simulink library "HybridFEMLibrary"  (Simulink 7.0)
undefined symbols (not defined in the file or in its folder): Alpham, DiscIntNeverNeededParam, Elements, gamma1, gamma2, Integrator, Interpolations, sample, SampleRate
(part 1 of 2)
settings Model: Creator=Tommy  LastModifiedBy=Tommy

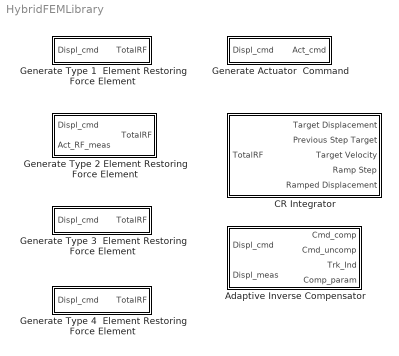
== system HybridFEMLibrary ==
  Adaptive Inverse Compensator : Subsystem
      mask Type: AIC
      mask Description: Adaptive Inverse Compensator produces a compensated command due to actuator delay.  Outputs the compensated and uncompensated response along with a tracking indicator and evolutionary compensation parameter.
  CR Integrator : Subsystem
      mask Type: CR Integrator
      mask Description: CR Integrator for performing the integration of the effective force history to produce the displacement and velocity commands for each time step.  Also combines the restoring force vectors and calculates the next step acceleration.
  Generate Actuator  Command : Subsystem  mask(Generate Actuator Command){id=0}
      mask prompts: id "Element ID"
      mask help:
      | Generates the local actuator command for the element referenced with Element ID
      |
      | Enter the ID for this element corresponding with the input configuration file
  Generate Type 1  Element Restoring Force Element : Subsystem  TreatAsAtomicUnit=on  SystemSampleTime=SampleRate  mask(Generate Type 1 Element Restoring Force){id=32}
      mask prompts: id "Element ID"
      mask help:
      | Generates the Restoring Force vector for a Type 1 Element
      |
      | Enter the ID for this element corresponding with the input configuration file
  Generate Type 2 Element Restoring Force Element : Subsystem  mask(Generate Type 2 Element Restoring Force){id=3, simulation=on}
      mask prompts: id "Element ID"; simulation "Experiment Mode"
      mask help:
      | Generates the Restoring Force vector for a Type 2 Element
      |
      | Enter the ID for this element corresponding with the input configuration file
      |
      | Check the "Experiment Mode" box to activate the Act_RF_meas input.
      | Connect the Actuator Restoring Force feedback to the input.
  Generate Type 3  Element Restoring Force Element : Subsystem  TreatAsAtomicUnit=on  SystemSampleTime=SampleRate  mask(Generate Type 3 Element Restoring Force){id=1}
      mask prompts: id "Element ID"
      mask help:
      | Generates the Restoring Force vector for a Type 3 Element
      |
      | Enter the ID for this element corresponding with the input configuration file
  Generate Type 4  Element Restoring Force Element : Subsystem  TreatAsAtomicUnit=on  SystemSampleTime=SampleRate  mask(Generate Type 4 Element Restoring Force){id=35}
      mask prompts: id "Element ID"
      mask help:
      | Generates the Restoring Force vector for a Type 4 Element
      |
      | Enter the ID for this element corresponding with the input configuration file

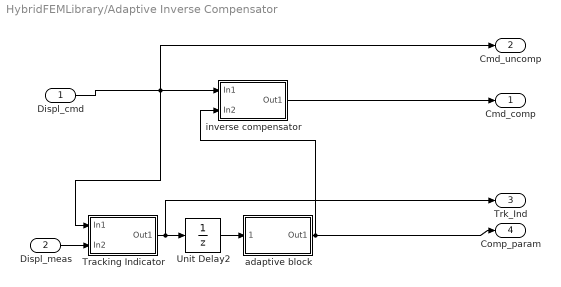
== system HybridFEMLibrary/Adaptive Inverse Compensator ==
  Displ_cmd : Inport  OutDataType=sfix(16)  OutScaling=2^0
  Displ_meas : Inport  Port=2  OutDataType=sfix(16)  OutScaling=2^0
  Tracking Indicator : Subsystem
  Unit Delay2 : UnitDelay  SampleTime=sample
  adaptive block : Subsystem
  inverse compensator : Subsystem
  Cmd_comp : Outport  OutDataType=sfix(16)  OutScaling=2^0
  Cmd_uncomp : Outport  Port=2  OutDataType=sfix(16)  OutScaling=2^0
  Trk_Ind : Outport  Port=3  OutDataType=sfix(16)  OutScaling=2^0
  Comp_param : Outport  Port=4  OutDataType=sfix(16)  OutScaling=2^0
  wires:
  inverse compensator/1(Out1) -> Cmd_comp/1
  adaptive block/1(Out1) -> inverse compensator/2(In2), Comp_param/1
  Tracking Indicator/1(Out1) -> Unit Delay2/1, Trk_Ind/1
  Unit Delay2/1 -> adaptive block/1(indicator)
  Displ_cmd/1 -> Cmd_uncomp/1, inverse compensator/1(In1), Tracking Indicator/1(In1)
  Displ_meas/1 -> Tracking Indicator/2(In2)

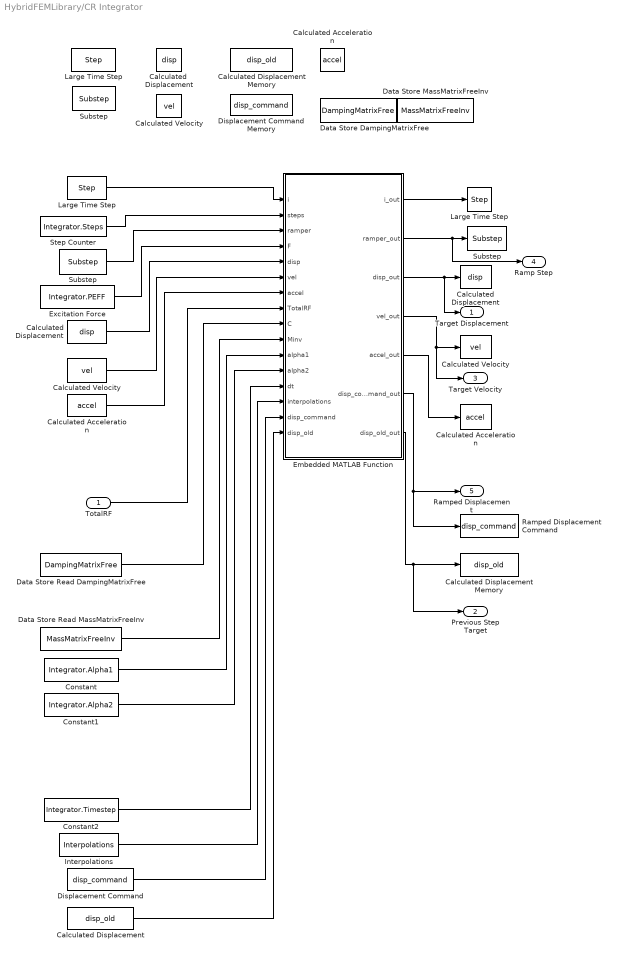
== system HybridFEMLibrary/CR Integrator ==
  TotalRF : Inport  OutDataType=sfix(16)  OutScaling=2^0
  " Calculated Acceleration" : DataStoreWrite  DataStoreName=accel  SampleTime=sample
  " Calculated Displacement" : DataStoreWrite  DataStoreName=disp  SampleTime=sample
  " Calculated Displacement Memory" : DataStoreWrite  DataStoreName=disp_old  SampleTime=sample
  " Calculated Velocity" : DataStoreWrite  DataStoreName=vel  SampleTime=sample
  " Large Time Step" : DataStoreWrite  DataStoreName=Step  SampleTime=sample
  " Substep" : DataStoreWrite  DataStoreName=Substep  SampleTime=sample
  Calculated Acceleration : DataStoreMemory  DataStoreName=accel  InitialValue=Integrator.Acceleration  OutDataType=sfix(16)  OutScaling=2^0
  Calculated Velocity : DataStoreMemory  DataStoreName=vel  InitialValue=Integrator.Velocity  OutDataType=sfix(16)  OutScaling=2^0
  Calculated  Displacement : DataStoreMemory  DataStoreName=disp  InitialValue=Integrator.Displacement  OutDataType=sfix(16)  OutScaling=2^0
  "Calculated Acceleration " : DataStoreRead  DataStoreName=accel  SampleTime=sample
  Calculated Displacement : DataStoreRead  DataStoreName=disp_old  SampleTime=sample
  Calculated Displacement Memory : DataStoreMemory  DataStoreName=disp_old  InitialValue=Integrator.Displacement  OutDataType=sfix(16)  OutScaling=2^0
  "Calculated Displacement " : DataStoreRead  DataStoreName=disp  SampleTime=sample
  "Calculated Velocity " : DataStoreRead  DataStoreName=vel  SampleTime=sample
  Constant : Constant  Value=Integrator.Alpha1  OutDataType=sfix(16)  OutScaling=2^0
  Constant1 : Constant  Value=Integrator.Alpha2  OutDataType=sfix(16)  OutScaling=2^0
  Constant2 : Constant  Value=Integrator.Timestep  OutDataType=sfix(16)  OutScaling=2^0
  Data Store DampingMatrixFree : DataStoreMemory  DataStoreName=DampingMatrixFree  InitialValue=Structure.DampingMatrixFree  OutDataType=sfix(16)  OutScaling=2^0
  Data Store MassMatrixFreeInv : DataStoreMemory  DataStoreName=MassMatrixFreeInv  InitialValue=Structure.MassMatrixFreeInv  OutDataType=sfix(16)  OutScaling=2^0
  Data Store Read DampingMatrixFree : DataStoreRead  DataStoreName=DampingMatrixFree  SampleTime=sample
  Data Store Read MassMatrixFreeInv : DataStoreRead  DataStoreName=MassMatrixFreeInv  SampleTime=sample
  Displacement Command Memory : DataStoreMemory  DataStoreName=disp_command  InitialValue=Integrator.Displacement  OutDataType=sfix(16)  OutScaling=2^0
  "Displacement Command " : DataStoreRead  DataStoreName=disp_command  SampleTime=sample
  Embedded MATLAB Function : Stateflow chart
  Excitation Force : Constant  Value=Integrator.PEFF  OutDataType=sfix(16)  OutScaling=2^0
  Interpolations : Constant  Value=Interpolations  OutDataType=sfix(16)  OutScaling=2^0  SampleTime=sample
  Large Time Step : DataStoreMemory  DataStoreName=Step  OutDataType=sfix(16)  OutScaling=2^0
  "Large Time Step " : DataStoreRead  DataStoreName=Step  SampleTime=sample
  Ramped Displacement Command : DataStoreWrite  DataStoreName=disp_command  SampleTime=sample
  Step Counter : Constant  Value=Integrator.Steps  OutDataType=sfix(16)  OutScaling=2^0  SampleTime=sample
  Substep : DataStoreMemory  DataStoreName=Substep  InitialValue=1  OutDataType=sfix(16)  OutScaling=2^0
  "Substep " : DataStoreRead  DataStoreName=Substep  SampleTime=sample
  Target Displacement : Outport  OutDataType=sfix(16)  OutScaling=2^0
  Previous Step Target : Outport  Port=2  OutDataType=sfix(16)  OutScaling=2^0
  Target Velocity : Outport  Port=3  OutDataType=sfix(16)  OutScaling=2^0
  Ramp Step : Outport  Port=4  OutDataType=sfix(16)  OutScaling=2^0
  Ramped Displacement : Outport  Port=5  OutDataType=sfix(16)  OutScaling=2^0
  wires:
  Excitation Force/1 -> Embedded MATLAB Function/4(F)
  Calculated Displacement/1 -> Embedded MATLAB Function/16(disp_old)
  "Displacement Command "/1 -> Embedded MATLAB Function/15(disp_command)
  "Calculated Acceleration "/1 -> Embedded MATLAB Function/7(accel)
  "Calculated Velocity "/1 -> Embedded MATLAB Function/6(vel)
  "Calculated Displacement "/1 -> Embedded MATLAB Function/5(disp)
  "Substep "/1 -> Embedded MATLAB Function/3(ramper)
  Embedded MATLAB Function/7(disp_old_out) -> Previous Step Target/1, " Calculated Displacement Memory"/1
  Embedded MATLAB Function/5(accel_out) -> " Calculated Acceleration"/1
  Embedded MATLAB Function/3(disp_out) -> " Calculated Displacement"/1, Target Displacement/1
  Embedded MATLAB Function/2(ramper_out) -> Ramp Step/1, " Substep"/1
  Embedded MATLAB Function/1(i_out) -> " Large Time Step"/1
  Constant1/1 -> Embedded MATLAB Function/12(alpha2)
  Constant/1 -> Embedded MATLAB Function/11(alpha1)
  Step Counter/1 -> Embedded MATLAB Function/2(steps)
  Constant2/1 -> Embedded MATLAB Function/13(dt)
  TotalRF/1 -> Embedded MATLAB Function/8(TotalRF)
  Embedded MATLAB Function/6(disp_command_out) -> Ramped Displacement Command/1, Ramped Displacement/1
  Embedded MATLAB Function/4(vel_out) -> " Calculated Velocity"/1, Target Velocity/1
  Interpolations/1 -> Embedded MATLAB Function/14(interpolations)
  Data Store Read MassMatrixFreeInv/1 -> Embedded MATLAB Function/10(Minv)
  Data Store Read DampingMatrixFree/1 -> Embedded MATLAB Function/9(C)
  "Large Time Step "/1 -> Embedded MATLAB Function/1(i)

== system HybridFEMLibrary/Generate Actuator  Command ==
  Displ_cmd : Inport  OutDataType=sfix(16)  OutScaling=2^0
  Generate Actuator Command : Stateflow chart
  Type 2 Element : Subsystem  mask(Element Type 2){id=3}
      mask prompts: id "Element ID:"
      mask help: Enter the ID for this element corresponding with the input configuration file
  Act_cmd : Outport  OutDataType=sfix(16)  OutScaling=2^0
  wires:
  Generate Actuator Command/1(Command) -> Act_cmd/1
  Type 2 Element/1(Element) -> Generate Actuator Command/1(Element)
  Displ_cmd/1 -> Generate Actuator Command/2(Displacement)

== system HybridFEMLibrary/Generate Type 1  Element Restoring Force Element ==
  Displ_cmd : Inport  OutDataType=sfix(16)  OutScaling=2^0
  "Type 1 Element " : Subsystem  mask(Element Type 1){id=id}
      mask prompts: id "Element ID:"
      mask help: Enter the ID for this element corresponding with the input configuration file
  Type 1 Element RF : Stateflow chart  TreatAsAtomicUnit=on  SystemSampleTime=SampleRate
  TotalRF : Outport  OutDataType=sfix(16)  OutScaling=2^0
  wires:
  Type 1 Element RF/1(TotalRF) -> TotalRF/1
  Displ_cmd/1 -> Type 1 Element RF/2(Displacement)
  "Type 1 Element "/1(Element) -> Type 1 Element RF/1(Element)

== system HybridFEMLibrary/Generate Type 2 Element Restoring Force Element ==
  Displ_cmd : Inport  OutDataType=sfix(16)  OutScaling=2^0
  Act_RF_meas : Inport  Port=2  OutDataType=sfix(16)  OutScaling=2^0
  Constant1 : Constant  Value=simulation  OutDataType=sfix(16)  OutScaling=2^0
  Type 2 Element : Subsystem  mask(Element Type 2){id=id}
      mask prompts: id "Element ID:"
      mask help: Enter the ID for this element corresponding with the input configuration file
  Type 2 Element RF : Stateflow chart
  TotalRF : Outport  OutDataType=sfix(16)  OutScaling=2^0
  wires:
  Type 2 Element/1(Element) -> Type 2 Element RF/1(Element)
  Act_RF_meas/1 -> Type 2 Element RF/3(ActuatorRF)
  Type 2 Element RF/1(TotalRF) -> TotalRF/1
  Displ_cmd/1 -> Type 2 Element RF/2(Displacement)
  Constant1/1 -> Type 2 Element RF/4(simulation)

== system HybridFEMLibrary/Generate Type 3  Element Restoring Force Element ==
  Displ_cmd : Inport  OutDataType=sfix(16)  OutScaling=2^0
  "Type 3 Element " : Subsystem  mask(Element Type 3){id=id}
      mask prompts: id "Element ID:"
      mask help: Enter the ID for this element corresponding with the input configuration file
  Type 3 Element RF : Stateflow chart  TreatAsAtomicUnit=on  SystemSampleTime=SampleRate
  TotalRF : Outport  OutDataType=sfix(16)  OutScaling=2^0
  wires:
  Displ_cmd/1 -> Type 3 Element RF/6(Displacement)
  "Type 3 Element "/1(Element) -> Type 3 Element RF/1(Element)
  Type 3 Element RF/1(TotalRF) -> TotalRF/1
  "Type 3 Element "/2(a1) -> Type 3 Element RF/2(a1)
  "Type 3 Element "/3(a2) -> Type 3 Element RF/3(a2)
  "Type 3 Element "/4(pmx) -> Type 3 Element RF/4(pmx)
  "Type 3 Element "/5(bmy) -> Type 3 Element RF/5(bmy_init)

== system HybridFEMLibrary/Generate Type 4  Element Restoring Force Element ==
  Displ_cmd : Inport  OutDataType=sfix(16)  OutScaling=2^0
  "Type 4 Element " : Subsystem  mask(Element Type 4){id=id}
      mask prompts: id "Element ID:"
      mask help: Enter the ID for this element corresponding with the input configuration file
  Type 4 Element RF : Stateflow chart  TreatAsAtomicUnit=on  SystemSampleTime=SampleRate
  TotalRF : Outport  OutDataType=sfix(16)  OutScaling=2^0
  wires:
  "Type 4 Element "/1(Element) -> Type 4 Element RF/1(Element)
  Type 4 Element RF/1(TotalRF) -> TotalRF/1
  Displ_cmd/1 -> Type 4 Element RF/2(Displacement)

== system HybridFEMLibrary/Adaptive Inverse Compensator/Tracking Indicator ==
  note: dc
  note: dm
  note: A
  note: TA
  note: TI
  In1 : Inport  OutDataType=sfix(16)  OutScaling=2^0
  In2 : Inport  Port=2  OutDataType=sfix(16)  OutScaling=2^0
  A : Subsystem
  Gain : Gain  Gain=0.5  ParameterDataType=sfix(16)  ParameterScaling=2^0  OutDataType=sfix(16)  OutScaling=2^0
  Scope : Scope
      settings: SaveName=ScopeData4
  Sum : Sum  Inputs=|+-  OutDataType=sfix(16)  OutScaling=2^0
  TA : Subsystem
  Out1 : Outport  OutDataType=sfix(16)  OutScaling=2^0
  wires:
  In2/1 -> A/2(In2), TA/2(In2)
  In1/1 -> A/1(In1), TA/1(In1)
  TA/1(Out1) -> Sum/2
  A/1(Out1) -> Sum/1
  Sum/1 -> Gain/1
  Gain/1 -> Out1/1, Scope/1

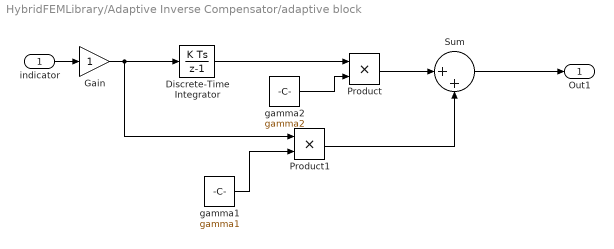
== system HybridFEMLibrary/Adaptive Inverse Compensator/adaptive block ==
  indicator : Inport  OutDataType=sfix(16)  OutScaling=2^0
  Discrete-Time Integrator : DiscreteIntegrator  SampleTime=sample  OutDataType=sfix(16)  OutScaling=2^0  ICPrevOutput=DiscIntNeverNeededParam  ICPrevScaledInput=DiscIntNeverNeededParam
  Gain : Gain  ParameterDataType=sfix(16)  ParameterScaling=2^0  OutDataType=sfix(16)  OutScaling=2^0
  Product : Product  OutDataType=sfix(16)  OutScaling=2^0  RndMeth=Zero
  Product1 : Product  OutDataType=sfix(16)  OutScaling=2^0  RndMeth=Zero
  Sum : Sum  Inputs=|++  OutDataType=sfix(16)  OutScaling=2^0
  gamma1 : Constant  Value=gamma1  OutDataType=sfix(16)  OutScaling=2^0
  gamma2 : Constant  Value=gamma2  OutDataType=sfix(16)  OutScaling=2^0
  Out1 : Outport  OutDataType=sfix(16)  OutScaling=2^0
  wires:
  Discrete-Time Integrator/1 -> Product/1
  gamma2/1 -> Product/2
  gamma1/1 -> Product1/2
  Product/1 -> Sum/1
  Sum/1 -> Out1/1
  indicator/1 -> Gain/1
  Product1/1 -> Sum/2
  Gain/1 -> Discrete-Time Integrator/1, Product1/1

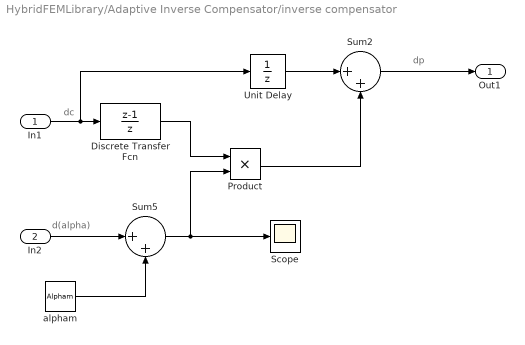
== system HybridFEMLibrary/Adaptive Inverse Compensator/inverse compensator ==
  note: dp
  note: d(alpha)
  note: dc
  In1 : Inport  OutDataType=sfix(16)  OutScaling=2^0
  In2 : Inport  Port=2  OutDataType=sfix(16)  OutScaling=2^0
  Discrete Transfer Fcn : DiscreteTransferFcn  Numerator=[1 -1]  Denominator=[1 0]  SampleTime=sample
  Product : Product  OutDataType=sfix(16)  OutScaling=2^0  RndMeth=Zero
  Scope : Scope
  Sum2 : Sum  Inputs=|++  OutDataType=sfix(16)  OutScaling=2^0
  Sum5 : Sum  Inputs=|++  OutDataType=sfix(16)  OutScaling=2^0
  Unit Delay : UnitDelay  SampleTime=sample
  alpham : Constant  Value=Alpham  OutDataType=sfix(16)  OutScaling=2^0
  Out1 : Outport  OutDataType=sfix(16)  OutScaling=2^0
  wires:
  Sum2/1 -> Out1/1
  Product/1 -> Sum2/2
  Unit Delay/1 -> Sum2/1
  Sum5/1 -> Scope/1, Product/2
  Discrete Transfer Fcn/1 -> Product/1
  alpham/1 -> Sum5/2
  In2/1 -> Sum5/1
  In1/1 -> Unit Delay/1, Discrete Transfer Fcn/1

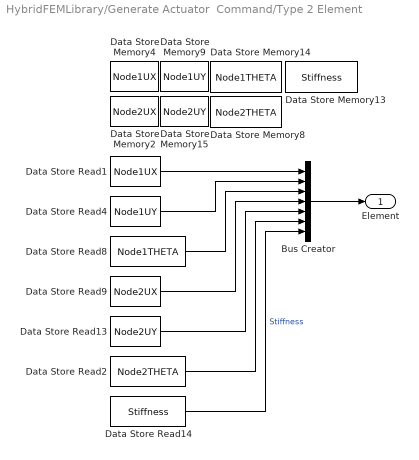
== system HybridFEMLibrary/Generate Actuator  Command/Type 2 Element ==
  Bus Creator : BusCreator  Inputs=7
  Data Store Memory13 : DataStoreMemory  DataStoreName=Stiffness  InitialValue=Elements{id}.Stiffness  OutDataType=sfix(16)  OutScaling=2^0
  Data Store Memory14 : DataStoreMemory  DataStoreName=Node1THETA  InitialValue=Elements{id}.Nodes(1).THETA  OutDataType=sfix(16)  OutScaling=2^0
  Data Store Memory15 : DataStoreMemory  DataStoreName=Node2UY  InitialValue=Elements{id}.Nodes(2).UY  OutDataType=sfix(16)  OutScaling=2^0
  Data Store Memory2 : DataStoreMemory  DataStoreName=Node2UX  InitialValue=Elements{id}.Nodes(2).UX  OutDataType=sfix(16)  OutScaling=2^0
  Data Store Memory4 : DataStoreMemory  DataStoreName=Node1UX  InitialValue=Elements{id}.Nodes(1).UX  OutDataType=sfix(16)  OutScaling=2^0
  Data Store Memory8 : DataStoreMemory  DataStoreName=Node2THETA  InitialValue=Elements{id}.Nodes(2).THETA  OutDataType=sfix(16)  OutScaling=2^0
  Data Store Memory9 : DataStoreMemory  DataStoreName=Node1UY  InitialValue=Elements{id}.Nodes(1).UY  OutDataType=sfix(16)  OutScaling=2^0
  Data Store Read1 : DataStoreRead  DataStoreName=Node1UX  SampleTime=-1
  Data Store Read13 : DataStoreRead  DataStoreName=Node2UY  SampleTime=-1
  Data Store Read14 : DataStoreRead  DataStoreName=Stiffness  SampleTime=-1
  Data Store Read2 : DataStoreRead  DataStoreName=Node2THETA  SampleTime=-1
  Data Store Read4 : DataStoreRead  DataStoreName=Node1UY  SampleTime=-1
  Data Store Read8 : DataStoreRead  DataStoreName=Node1THETA  SampleTime=-1
  Data Store Read9 : DataStoreRead  DataStoreName=Node2UX  SampleTime=-1
  Element : Outport  OutDataType=sfix(16)  OutScaling=2^0
  wires:
  Bus Creator/1 -> Element/1
  Data Store Read14/1 -> Bus Creator/7  "Stiffness"
  Data Store Read2/1 -> Bus Creator/6
  Data Store Read13/1 -> Bus Creator/5
  Data Store Read9/1 -> Bus Creator/4
  Data Store Read8/1 -> Bus Creator/3
  Data Store Read4/1 -> Bus Creator/2
  Data Store Read1/1 -> Bus Creator/1

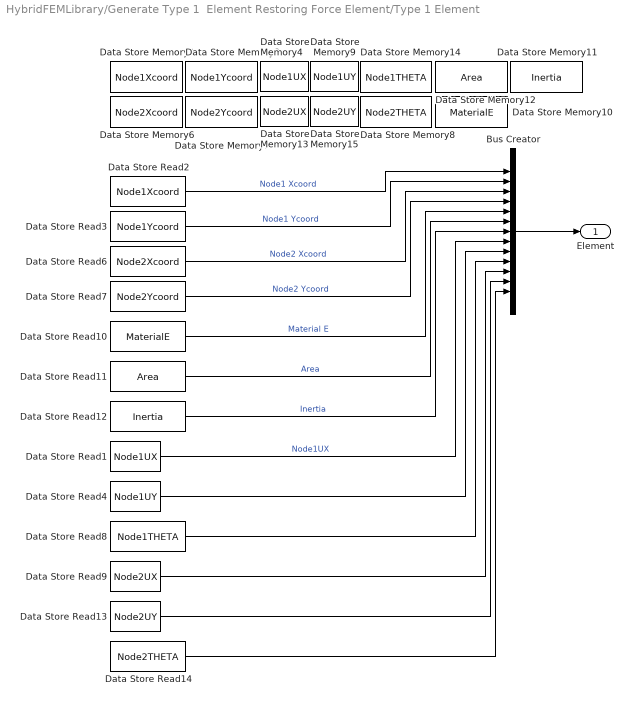
== system HybridFEMLibrary/Generate Type 1  Element Restoring Force Element/Type 1 Element  ==
  Bus Creator : BusCreator  Inputs=13
  Data Store Memory10 : DataStoreMemory  DataStoreName=MaterialE  InitialValue=Elements{id}.Material(1).E  OutDataType=sfix(16)  OutScaling=2^0
  Data Store Memory11 : DataStoreMemory  DataStoreName=Inertia  InitialValue=Elements{id}.Inertia  OutDataType=sfix(16)  OutScaling=2^0
  Data Store Memory12 : DataStoreMemory  DataStoreName=Area  InitialValue=Elements{id}.Area  OutDataType=sfix(16)  OutScaling=2^0
  Data Store Memory13 : DataStoreMemory  DataStoreName=Node2UX  InitialValue=Elements{id}.Nodes(2).UX  OutDataType=sfix(16)  OutScaling=2^0
  Data Store Memory14 : DataStoreMemory  DataStoreName=Node1THETA  InitialValue=Elements{id}.Nodes(1).THETA  OutDataType=sfix(16)  OutScaling=2^0
  Data Store Memory15 : DataStoreMemory  DataStoreName=Node2UY  InitialValue=Elements{id}.Nodes(2).UY  OutDataType=sfix(16)  OutScaling=2^0
  Data Store Memory2 : DataStoreMemory  DataStoreName=Node1Xcoord  InitialValue=Elements{id}.Nodes(1).Xcoord  OutDataType=sfix(16)  OutScaling=2^0
  Data Store Memory3 : DataStoreMemory  DataStoreName=Node1Ycoord  InitialValue=Elements{id}.Nodes(1).Ycoord  OutDataType=sfix(16)  OutScaling=2^0
  Data Store Memory4 : DataStoreMemory  DataStoreName=Node1UX  InitialValue=Elements{id}.Nodes(1).UX  OutDataType=sfix(16)  OutScaling=2^0
  Data Store Memory6 : DataStoreMemory  DataStoreName=Node2Xcoord  InitialValue=Elements{id}.Nodes(2).Xcoord  OutDataType=sfix(16)  OutScaling=2^0
  Data Store Memory7 : DataStoreMemory  DataStoreName=Node2Ycoord  InitialValue=Elements{id}.Nodes(2).Ycoord  OutDataType=sfix(16)  OutScaling=2^0
  Data Store Memory8 : DataStoreMemory  DataStoreName=Node2THETA  InitialValue=Elements{id}.Nodes(2).THETA  OutDataType=sfix(16)  OutScaling=2^0
  Data Store Memory9 : DataStoreMemory  DataStoreName=Node1UY  InitialValue=Elements{id}.Nodes(1).UY  OutDataType=sfix(16)  OutScaling=2^0
  Data Store Read1 : DataStoreRead  DataStoreName=Node1UX  SampleTime=-1
  Data Store Read10 : DataStoreRead  DataStoreName=MaterialE  SampleTime=-1
  Data Store Read11 : DataStoreRead  DataStoreName=Area  SampleTime=-1
  Data Store Read12 : DataStoreRead  DataStoreName=Inertia  SampleTime=-1
  Data Store Read13 : DataStoreRead  DataStoreName=Node2UY  SampleTime=-1
  Data Store Read14 : DataStoreRead  DataStoreName=Node2THETA  SampleTime=-1
  Data Store Read2 : DataStoreRead  DataStoreName=Node1Xcoord  SampleTime=-1
  Data Store Read3 : DataStoreRead  DataStoreName=Node1Ycoord  SampleTime=-1
  Data Store Read4 : DataStoreRead  DataStoreName=Node1UY  SampleTime=-1
  Data Store Read6 : DataStoreRead  DataStoreName=Node2Xcoord  SampleTime=-1
  Data Store Read7 : DataStoreRead  DataStoreName=Node2Ycoord  SampleTime=-1
  Data Store Read8 : DataStoreRead  DataStoreName=Node1THETA  SampleTime=-1
  Data Store Read9 : DataStoreRead  DataStoreName=Node2UX  SampleTime=-1
  Element : Outport  OutDataType=sfix(16)  OutScaling=2^0
  wires:
  Bus Creator/1 -> Element/1
  Data Store Read12/1 -> Bus Creator/7  "Inertia"
  Data Store Read11/1 -> Bus Creator/6  "Area"
  Data Store Read10/1 -> Bus Creator/5  "Material E"
  Data Store Read7/1 -> Bus Creator/4  "Node2 Ycoord"
  Data Store Read6/1 -> Bus Creator/3  "Node2 Xcoord"
  Data Store Read3/1 -> Bus Creator/2  "Node1 Ycoord"
  Data Store Read2/1 -> Bus Creator/1  "Node1 Xcoord"
  Data Store Read1/1 -> Bus Creator/8  "Node1UX"
  Data Store Read4/1 -> Bus Creator/9
  Data Store Read8/1 -> Bus Creator/10
  Data Store Read9/1 -> Bus Creator/11
  Data Store Read13/1 -> Bus Creator/12
  Data Store Read14/1 -> Bus Creator/13

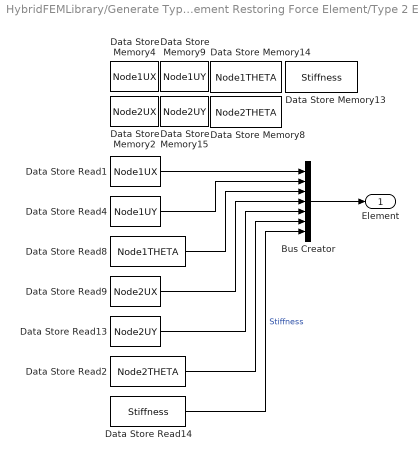
== system HybridFEMLibrary/Generate Type 2 Element Restoring Force Element/Type 2 Element ==
  Bus Creator : BusCreator  Inputs=7
  Data Store Memory13 : DataStoreMemory  DataStoreName=Stiffness  InitialValue=Elements{id}.Stiffness  OutDataType=sfix(16)  OutScaling=2^0
  Data Store Memory14 : DataStoreMemory  DataStoreName=Node1THETA  InitialValue=Elements{id}.Nodes(1).THETA  OutDataType=sfix(16)  OutScaling=2^0
  Data Store Memory15 : DataStoreMemory  DataStoreName=Node2UY  InitialValue=Elements{id}.Nodes(2).UY  OutDataType=sfix(16)  OutScaling=2^0
  Data Store Memory2 : DataStoreMemory  DataStoreName=Node2UX  InitialValue=Elements{id}.Nodes(2).UX  OutDataType=sfix(16)  OutScaling=2^0
  Data Store Memory4 : DataStoreMemory  DataStoreName=Node1UX  InitialValue=Elements{id}.Nodes(1).UX  OutDataType=sfix(16)  OutScaling=2^0
  Data Store Memory8 : DataStoreMemory  DataStoreName=Node2THETA  InitialValue=Elements{id}.Nodes(2).THETA  OutDataType=sfix(16)  OutScaling=2^0
  Data Store Memory9 : DataStoreMemory  DataStoreName=Node1UY  InitialValue=Elements{id}.Nodes(1).UY  OutDataType=sfix(16)  OutScaling=2^0
  Data Store Read1 : DataStoreRead  DataStoreName=Node1UX  SampleTime=-1
  Data Store Read13 : DataStoreRead  DataStoreName=Node2UY  SampleTime=-1
  Data Store Read14 : DataStoreRead  DataStoreName=Stiffness  SampleTime=-1
  Data Store Read2 : DataStoreRead  DataStoreName=Node2THETA  SampleTime=-1
  Data Store Read4 : DataStoreRead  DataStoreName=Node1UY  SampleTime=-1
  Data Store Read8 : DataStoreRead  DataStoreName=Node1THETA  SampleTime=-1
  Data Store Read9 : DataStoreRead  DataStoreName=Node2UX  SampleTime=-1
  Element : Outport  OutDataType=sfix(16)  OutScaling=2^0
  wires:
  Data Store Read1/1 -> Bus Creator/1
  Data Store Read4/1 -> Bus Creator/2
  Data Store Read8/1 -> Bus Creator/3
  Data Store Read9/1 -> Bus Creator/4
  Data Store Read13/1 -> Bus Creator/5
  Data Store Read2/1 -> Bus Creator/6
  Data Store Read14/1 -> Bus Creator/7  "Stiffness"
  Bus Creator/1 -> Element/1

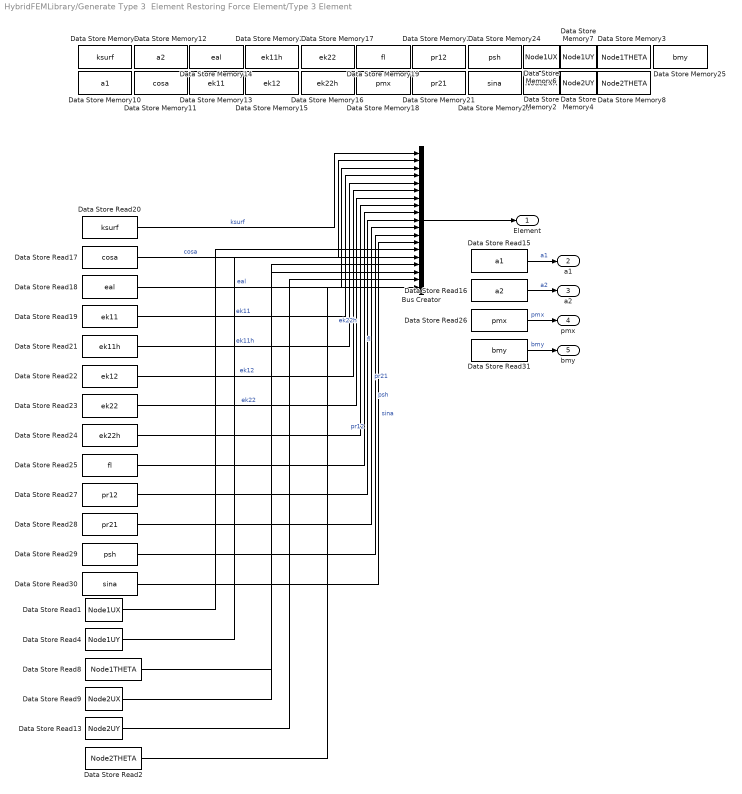
== system HybridFEMLibrary/Generate Type 3  Element Restoring Force Element/Type 3 Element  ==
  Bus Creator : BusCreator  Inputs=19
  Data Store Memory10 : DataStoreMemory  DataStoreName=a1  InitialValue=Elements{id}.a1  OutDataType=sfix(16)  OutScaling=2^0
  Data Store Memory11 : DataStoreMemory  DataStoreName=cosa  InitialValue=Elements{id}.cosa  OutDataType=sfix(16)  OutScaling=2^0
  Data Store Memory12 : DataStoreMemory  DataStoreName=a2  InitialValue=Elements{id}.a2  OutDataType=sfix(16)  OutScaling=2^0
  Data Store Memory13 : DataStoreMemory  DataStoreName=ek11  InitialValue=Elements{id}.ek11  OutDataType=sfix(16)  OutScaling=2^0
  Data Store Memory14 : DataStoreMemory  DataStoreName=eal  InitialValue=Elements{id}.eal  OutDataType=sfix(16)  OutScaling=2^0
  Data Store Memory15 : DataStoreMemory  DataStoreName=ek12  InitialValue=Elements{id}.ek12  OutDataType=sfix(16)  OutScaling=2^0
  Data Store Memory16 : DataStoreMemory  DataStoreName=ek22h  InitialValue=Elements{id}.ek22h  OutDataType=sfix(16)  OutScaling=2^0
  Data Store Memory17 : DataStoreMemory  DataStoreName=ek22  InitialValue=Elements{id}.ek22  OutDataType=sfix(16)  OutScaling=2^0
  Data Store Memory18 : DataStoreMemory  DataStoreName=pmx  InitialValue=Elements{id}.pmx  OutDataType=sfix(16)  OutScaling=2^0
  Data Store Memory19 : DataStoreMemory  DataStoreName=fl  InitialValue=Elements{id}.fl  OutDataType=sfix(16)  OutScaling=2^0
  Data Store Memory2 : DataStoreMemory  DataStoreName=Node2UX  InitialValue=Elements{id}.Nodes(2).UX  OutDataType=sfix(16)  OutScaling=2^0
  Data Store Memory20 : DataStoreMemory  DataStoreName=ek11h  InitialValue=Elements{id}.ek11h  OutDataType=sfix(16)  OutScaling=2^0
  Data Store Memory21 : DataStoreMemory  DataStoreName=pr21  InitialValue=Elements{id}.pr21  OutDataType=sfix(16)  OutScaling=2^0
  Data Store Memory22 : DataStoreMemory  DataStoreName=pr12  InitialValue=Elements{id}.pr12  OutDataType=sfix(16)  OutScaling=2^0
  Data Store Memory23 : DataStoreMemory  DataStoreName=sina  InitialValue=Elements{id}.sina  OutDataType=sfix(16)  OutScaling=2^0
  Data Store Memory24 : DataStoreMemory  DataStoreName=psh  InitialValue=Elements{id}.psh  OutDataType=sfix(16)  OutScaling=2^0
  Data Store Memory25 : DataStoreMemory  DataStoreName=bmy  InitialValue=Elements{id}.bmy  OutDataType=sfix(16)  OutScaling=2^0
  Data Store Memory3 : DataStoreMemory  DataStoreName=Node1THETA  InitialValue=Elements{id}.Nodes(1).THETA  OutDataType=sfix(16)  OutScaling=2^0
  Data Store Memory4 : DataStoreMemory  DataStoreName=Node2UY  InitialValue=Elements{id}.Nodes(2).UY  OutDataType=sfix(16)  OutScaling=2^0
  Data Store Memory6 : DataStoreMemory  DataStoreName=Node1UX  InitialValue=Elements{id}.Nodes(1).UX  OutDataType=sfix(16)  OutScaling=2^0
  Data Store Memory7 : DataStoreMemory  DataStoreName=Node1UY  InitialValue=Elements{id}.Nodes(1).UY  OutDataType=sfix(16)  OutScaling=2^0
  Data Store Memory8 : DataStoreMemory  DataStoreName=Node2THETA  InitialValue=Elements{id}.Nodes(2).THETA  OutDataType=sfix(16)  OutScaling=2^0
  Data Store Memory9 : DataStoreMemory  DataStoreName=ksurf  InitialValue=Elements{id}.ksurf  OutDataType=sfix(16)  OutScaling=2^0
  Data Store Read1 : DataStoreRead  DataStoreName=Node1UX  SampleTime=-1
  Data Store Read13 : DataStoreRead  DataStoreName=Node2UY  SampleTime=-1
  Data Store Read15 : DataStoreRead  DataStoreName=a1  SampleTime=-1
  Data Store Read16 : DataStoreRead  DataStoreName=a2  SampleTime=-1
  Data Store Read17 : DataStoreRead  DataStoreName=cosa  SampleTime=-1
  Data Store Read18 : DataStoreRead  DataStoreName=eal  SampleTime=-1
  Data Store Read19 : DataStoreRead  DataStoreName=ek11  SampleTime=-1
  Data Store Read2 : DataStoreRead  DataStoreName=Node2THETA  SampleTime=-1
  Data Store Read20 : DataStoreRead  DataStoreName=ksurf  SampleTime=-1
  Data Store Read21 : DataStoreRead  DataStoreName=ek11h  SampleTime=-1
  Data Store Read22 : DataStoreRead  DataStoreName=ek12  SampleTime=-1
  Data Store Read23 : DataStoreRead  DataStoreName=ek22  SampleTime=-1
  Data Store Read24 : DataStoreRead  DataStoreName=ek22h  SampleTime=-1
  Data Store Read25 : DataStoreRead  DataStoreName=fl  SampleTime=-1
  Data Store Read26 : DataStoreRead  DataStoreName=pmx  SampleTime=-1
  Data Store Read27 : DataStoreRead  DataStoreName=pr12  SampleTime=-1
  Data Store Read28 : DataStoreRead  DataStoreName=pr21  SampleTime=-1
  Data Store Read29 : DataStoreRead  DataStoreName=psh  SampleTime=-1
  Data Store Read30 : DataStoreRead  DataStoreName=sina  SampleTime=-1
  Data Store Read31 : DataStoreRead  DataStoreName=bmy  SampleTime=-1
  Data Store Read4 : DataStoreRead  DataStoreName=Node1UY  SampleTime=-1
  Data Store Read8 : DataStoreRead  DataStoreName=Node1THETA  SampleTime=-1
  Data Store Read9 : DataStoreRead  DataStoreName=Node2UX  SampleTime=-1
  Element : Outport  OutDataType=sfix(16)  OutScaling=2^0
  a1 : Outport  Port=2  OutDataType=sfix(16)  OutScaling=2^0
  a2 : Outport  Port=3  OutDataType=sfix(16)  OutScaling=2^0
  pmx : Outport  Port=4  OutDataType=sfix(16)  OutScaling=2^0
  bmy : Outport  Port=5  OutDataType=sfix(16)  OutScaling=2^0
  wires:
  Data Store Read31/1 -> bmy/1  "bmy"
  Data Store Read26/1 -> pmx/1  "pmx"
  Data Store Read16/1 -> a2/1  "a2"
  Data Store Read15/1 -> a1/1  "a1"
  Data Store Read30/1 -> Bus Creator/13  "sina"
  Data Store Read29/1 -> Bus Creator/12  "psh"
  Data Store Read28/1 -> Bus Creator/11  "pr21"
  Data Store Read27/1 -> Bus Creator/10  "pr12"
  Data Store Read25/1 -> Bus Creator/9  "fl"
  Data Store Read24/1 -> Bus Creator/8  "ek22h"
  Data Store Read23/1 -> Bus Creator/7  "ek22"
  Data Store Read22/1 -> Bus Creator/6  "ek12"
  Data Store Read21/1 -> Bus Creator/5  "ek11h"
  Data Store Read19/1 -> Bus Creator/4  "ek11"
  Data Store Read18/1 -> Bus Creator/3  "eal"
  Data Store Read17/1 -> Bus Creator/2  "cosa"
  Data Store Read20/1 -> Bus Creator/1  "ksurf"
  Bus Creator/1 -> Element/1
  Data Store Read1/1 -> Bus Creator/14
  Data Store Read4/1 -> Bus Creator/15
  Data Store Read8/1 -> Bus Creator/16
  Data Store Read9/1 -> Bus Creator/17
  Data Store Read13/1 -> Bus Creator/18
  Data Store Read2/1 -> Bus Creator/19

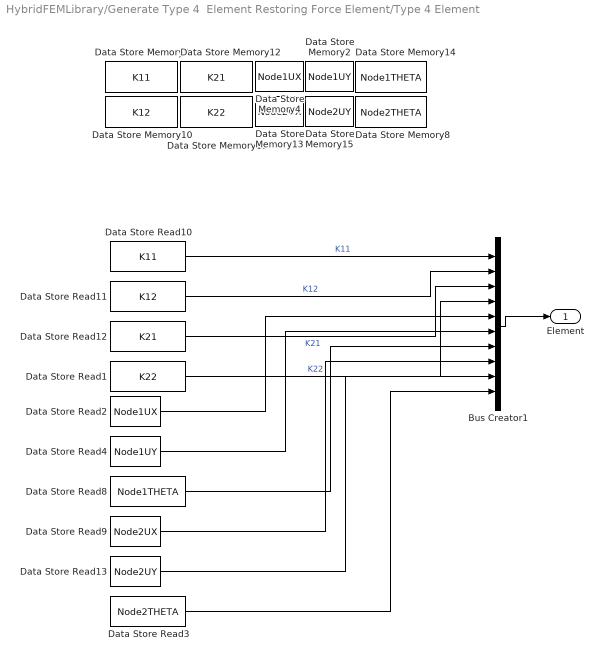
== system HybridFEMLibrary/Generate Type 4  Element Restoring Force Element/Type 4 Element  ==
  Bus Creator1 : BusCreator  Inputs=10
  Data Store Memory10 : DataStoreMemory  DataStoreName=K12  InitialValue=Elements{id}.K12  OutDataType=sfix(16)  OutScaling=2^0
  Data Store Memory11 : DataStoreMemory  DataStoreName=K22  InitialValue=Elements{id}.K22  OutDataType=sfix(16)  OutScaling=2^0
  Data Store Memory12 : DataStoreMemory  DataStoreName=K21  InitialValue=Elements{id}.K21  OutDataType=sfix(16)  OutScaling=2^0
  Data Store Memory13 : DataStoreMemory  DataStoreName=Node2UX  InitialValue=Elements{id}.Nodes(2).UX  OutDataType=sfix(16)  OutScaling=2^0
  Data Store Memory14 : DataStoreMemory  DataStoreName=Node1THETA  InitialValue=Elements{id}.Nodes(1).THETA  OutDataType=sfix(16)  OutScaling=2^0
  Data Store Memory15 : DataStoreMemory  DataStoreName=Node2UY  InitialValue=Elements{id}.Nodes(2).UY  OutDataType=sfix(16)  OutScaling=2^0
  Data Store Memory2 : DataStoreMemory  DataStoreName=Node1UY  InitialValue=Elements{id}.Nodes(1).UY  OutDataType=sfix(16)  OutScaling=2^0
  Data Store Memory4 : DataStoreMemory  DataStoreName=Node1UX  InitialValue=Elements{id}.Nodes(1).UX  OutDataType=sfix(16)  OutScaling=2^0
  Data Store Memory8 : DataStoreMemory  DataStoreName=Node2THETA  InitialValue=Elements{id}.Nodes(2).THETA  OutDataType=sfix(16)  OutScaling=2^0
  Data Store Memory9 : DataStoreMemory  DataStoreName=K11  InitialValue=Elements{id}.K11  OutDataType=sfix(16)  OutScaling=2^0
  Data Store Read1 : DataStoreRead  DataStoreName=K22  SampleTime=-1
  Data Store Read10 : DataStoreRead  DataStoreName=K11  SampleTime=-1
  Data Store Read11 : DataStoreRead  DataStoreName=K12  SampleTime=-1
  Data Store Read12 : DataStoreRead  DataStoreName=K21  SampleTime=-1
  Data Store Read13 : DataStoreRead  DataStoreName=Node2UY  SampleTime=-1
  Data Store Read2 : DataStoreRead  DataStoreName=Node1UX  SampleTime=-1
  Data Store Read3 : DataStoreRead  DataStoreName=Node2THETA  SampleTime=-1
  Data Store Read4 : DataStoreRead  DataStoreName=Node1UY  SampleTime=-1
  Data Store Read8 : DataStoreRead  DataStoreName=Node1THETA  SampleTime=-1
  Data Store Read9 : DataStoreRead  DataStoreName=Node2UX  SampleTime=-1
  Element : Outport  OutDataType=sfix(16)  OutScaling=2^0
  wires:
  Data Store Read3/1 -> Bus Creator1/10
  Data Store Read13/1 -> Bus Creator1/9
  Data Store Read9/1 -> Bus Creator1/8
  Data Store Read8/1 -> Bus Creator1/7
  Data Store Read4/1 -> Bus Creator1/6
  Data Store Read2/1 -> Bus Creator1/5
  Bus Creator1/1 -> Element/1
  Data Store Read10/1 -> Bus Creator1/1  "K11"
  Data Store Read11/1 -> Bus Creator1/2  "K12"
  Data Store Read12/1 -> Bus Creator1/3  "K21"
  Data Store Read1/1 -> Bus Creator1/4  "K22"

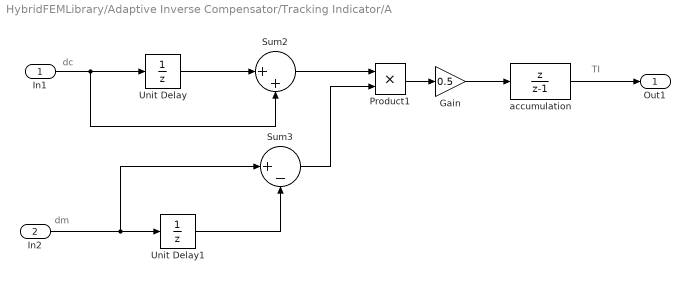
== system HybridFEMLibrary/Adaptive Inverse Compensator/Tracking Indicator/A ==
  note: dc
  note: dm
  note: TI
  In1 : Inport  OutDataType=sfix(16)  OutScaling=2^0
  In2 : Inport  Port=2  OutDataType=sfix(16)  OutScaling=2^0
  Gain : Gain  Gain=0.5  ParameterDataType=sfix(16)  ParameterScaling=2^0  OutDataType=sfix(16)  OutScaling=2^0
  Product1 : Product  OutDataType=sfix(16)  OutScaling=2^0  RndMeth=Zero
  Sum2 : Sum  Inputs=|++  OutDataType=sfix(16)  OutScaling=2^0
  Sum3 : Sum  Inputs=|+-  OutDataType=sfix(16)  OutScaling=2^0
  Unit Delay : UnitDelay  SampleTime=sample
  Unit Delay1 : UnitDelay  SampleTime=sample
  accumulation : DiscreteTransferFcn  Numerator=[1 0]  Denominator=[1 -1]  SampleTime=sample
  Out1 : Outport  OutDataType=sfix(16)  OutScaling=2^0
  wires:
  In1/1 -> Unit Delay/1, Sum2/2
  In2/1 -> Sum3/1, Unit Delay1/1
  Unit Delay/1 -> Sum2/1
  Unit Delay1/1 -> Sum3/2
  Sum2/1 -> Product1/1
  Sum3/1 -> Product1/2
  Product1/1 -> Gain/1
  Gain/1 -> accumulation/1
  accumulation/1 -> Out1/1

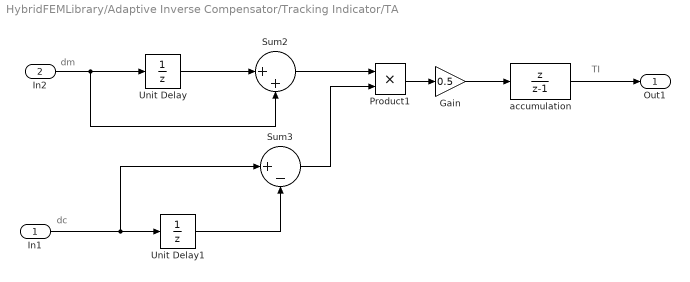
== system HybridFEMLibrary/Adaptive Inverse Compensator/Tracking Indicator/TA ==
  note: dm
  note: dc
  note: TI
  In1 : Inport  OutDataType=sfix(16)  OutScaling=2^0
  In2 : Inport  Port=2  OutDataType=sfix(16)  OutScaling=2^0
  Gain : Gain  Gain=0.5  ParameterDataType=sfix(16)  ParameterScaling=2^0  OutDataType=sfix(16)  OutScaling=2^0
  Product1 : Product  OutDataType=sfix(16)  OutScaling=2^0  RndMeth=Zero
  Sum2 : Sum  Inputs=|++  OutDataType=sfix(16)  OutScaling=2^0
  Sum3 : Sum  Inputs=|+-  OutDataType=sfix(16)  OutScaling=2^0
  Unit Delay : UnitDelay  SampleTime=sample
  Unit Delay1 : UnitDelay  SampleTime=sample
  accumulation : DiscreteTransferFcn  Numerator=[1 0]  Denominator=[1 -1]  SampleTime=sample
  Out1 : Outport  OutDataType=sfix(16)  OutScaling=2^0
  wires:
  In2/1 -> Unit Delay/1, Sum2/2
  In1/1 -> Sum3/1, Unit Delay1/1
  Unit Delay/1 -> Sum2/1
  Unit Delay1/1 -> Sum3/2
  Sum2/1 -> Product1/1
  Sum3/1 -> Product1/2
  Product1/1 -> Gain/1
  Gain/1 -> accumulation/1
  accumulation/1 -> Out1/1

== matlab function Generate Type 2 Element Restoring Force Element/Type 2 Element RF ==
  data: TotalRF output inherited; Element input inherited; Displacement input inherited; ActuatorRF input inherited; simulation input inherited; NumFreeDOF parameter inherited
% get restoring force for the element
% returns (6x1) restoring force vector of element in global coordinates
function TotalRF  = fcn(Element, Displacement, ActuatorRF, simulation, NumFreeDOF)

%% Input mapping
Node1UX = Element(1);
Node1UY = Element(2);
Node1THETA = Element(3);
Node2UX = Element(4);
Node2UY = Element(5);
Node2THETA = Element(6);
Stiffness = Element(7);

% Check if it is a simulation or using real RF
if (simulation == 0)
    % preset arrays
    SE = zeros(6,6);

    % Form Stiffness Matrix
    SE(1, 1) = Stiffness;
    SE(1, 4) = -Stiffness;
    SE(4, 4) = Stiffness;
    SE(4, 1) = SE(1,4);
    
    %create the displacement Ue (6x1) vector of the element in global coordinates
    Ue=zeros(6,1);
    dof=zeros(6,1);
    dof(1,1)=Node1UX;
    dof(2,1)=Node1UY;
    dof(3,1)=Node1THETA;
    dof(4,1)=Node2UX;
    dof(5,1)=Node2UY;
    dof(6,1)=Node2THETA;
    for i=1:6
        if dof(i,1)<=NumFreeDOF
            Ue(i,1)=Displacement(dof(i,1),1);
        end
    end
    RF = SE*Ue;  %resisting (6x1) resisting force vector of element in global coordinates
else
    RestoringForce = zeros(6,1);
    RestoringForce(1,1) = ActuatorRF;
    RestoringForce(4,1) = -ActuatorRF;
	RF = RestoringForce;
end

% Form total restoring force vector
TotalRF = zeros(NumFreeDOF, 1);
    
% Get element nodes to assemble in the structure restoring force vector
if Node1UX <= NumFreeDOF
    TotalRF(Node1UX, 1) = RF(1, 1);
end
if Node1UY <= NumFreeDOF
    TotalRF(Node1UY, 1) = RF(2, 1);
end
if Node1THETA <= NumFreeDOF
    TotalRF(Node1THETA, 1) = RF(3, 1);
end
if Node2UX <= NumFreeDOF
    TotalRF(Node2UX, 1) = RF(4, 1);
end
if Node2UY <= NumFreeDOF
    TotalRF(Node2UY, 1) = RF(5, 1);
end
if Node2THETA <= NumFreeDOF
    TotalRF(Node2THETA, 1) = RF(6, 1);
end

== matlab function CR Integrator/Embedded MATLAB Function ==
  data: i input inherited; steps input inherited; i_out output inherited; ramper_out output inherited; ramper input inherited; F input inherited; disp input inherited; vel input inherited; accel input inherited; TotalRF input inherited; C input inherited; Minv input inherited; disp_out output inherited; vel_out output inherited; accel_out output inherited; alpha1 input inherited; alpha2 input inherited; dt input inherited; interpolations input inherited; disp_command input inherited; disp_command_out output inherited; disp_old_out output inherited; disp_old input inherited
function [i_out,ramper_out,disp_out,vel_out,accel_out,disp_command_out,disp_old_out]  = fcn(i,steps,ramper,F,disp,vel,accel,TotalRF,C,Minv,alpha1,alpha2,dt,interpolations,disp_command,disp_old)

%% Main cycle occurs while the earthquake record isn't exhausted
if (i < steps-1)  
    %% First ramp of a new step, calculate displacement and velocity vectors
    if (ramper == 1)
        i = i + 1;                                  %increment to next step
        disp_old = disp;                            %save previous displacement
        disp = disp + dt*vel + alpha2*dt^2*accel;    %calculate next displacement vector
        vel = vel + alpha1*dt*accel;                 %calculate next velocity vector
    end
    
    %% Set ramped command vector
    disp_command_out = (disp - disp_old)/(interpolations) * (ramper) + disp_old;
    
    %% Check for the last ramper
    if (ramper == interpolations)
        ramper_out = 1;      

        % extrapolation
        %def = [disp(1); disp(2)-disp(1)];
        %def_old = [disp_old(1); disp_old(2)-disp_old(1)];
        %TotalRF = TotalRF + Kd*(def - def_old)/interpolations;
        
        accel = Minv*( F(i,:)' - C*vel - TotalRF ); %calculate new acceleration vector
        %accel = Minv*( F(i,:)' - C*vel - [TotalRF(1)-TotalRF(2);TotalRF(2)] ); %calculate new acceleration vector
    %% Ramp the command within the same earthquake step
    else
        ramper_out = ramper + 1;
    end
    
    %% Pass variables through to the next sample 
    i_out = i;                  %remember big time step
    disp_out = disp;            %remember displacement vector
    vel_out = vel;              %remember velocity vector
    accel_out = accel;          %remember acceleration vector
    disp_old_out = disp_old;    %remember previous displacement vector
          
%% Earthquake record exhausted so just set output = input for all variables
else
    i_out = i;
    ramper_out = ramper;
    disp_out = disp;    
    vel_out = vel;      
    accel_out = accel;
    disp_command_out = disp_command; 
    disp_old_out = disp_old;
end

== matlab function Generate Type 3 Element Restoring Force Element/Type 3 Element RF ==
  data: TotalRF output inherited; Element input inherited; a1 input inherited; a2 input inherited; pmx input inherited; bmy_init input inherited; Displacement input inherited; NumFreeDOF parameter inherited
% Get Restoring Force Type 3
function TotalRF  = fnc(Element, a1, a2, pmx, bmy_init, Displacement, NumFreeDOF)

persistent initialized;
persistent kody;
persistent bmep;
persistent bmel;
persistent bmtot;
persistent bbmy;
persistent dpr;
persistent bmy;
persistent ftot;
persistent pracn;
persistent pracp;
persistent prtot;
persistent sftot;
persistent Uprev;

%% Input mapping
ksurf = Element(1);
cosa = Element(2);
eal = Element(3);
ek11 = Element(4);
ek11h = Element(5);
ek12 = Element(6);
ek22 = Element(7);
ek22h = Element(8);
fl = Element(9);
pr12 = Element(10);
pr21 = Element(11);
psh = Element(12);
sina = Element(13);
Node1UX = Element(14);
Node1UY = Element(15);
Node1THETA = Element(16);
Node2UX = Element(17);
Node2UY = Element(18);
Node2THETA = Element(19);

if isempty(initialized)
    initialized = 1;
    kody = zeros(2,1);
    bmep = zeros(2,1); 
    bmel = zeros(2,1);
    bmtot = zeros(2,1);
    bbmy = 0;
    dpr = zeros(2,1);
    ftot = zeros(2,1);  
    pracn = zeros(2,1); 
    pracp = zeros(2,1);
    prtot = zeros(2,1);
    sftot = zeros(2,1); 
    Uprev = zeros(6,1);
    bmy = bmy_init;
end

%% Get the displacement Ue (6x1) vector of the element in global coordinates
Ue = zeros(6,1);
dof=zeros(6,1);
dof(1,1)=Node1UX;
dof(2,1)=Node1UY;
dof(3,1)=Node1THETA;
dof(4,1)=Node2UX;
dof(5,1)=Node2UY;
dof(6,1)=Node2THETA;
for i=1:6
    if dof(i,1)<=NumFreeDOF
        Ue(i,1)=Displacement(dof(i,1),1);
    end
end

%% Input of Drain State Determination Type 2 Element
ndof=6;  %the element has 6 dofs
ddise=Ue-Uprev;  %the incremental displacement vector ddise of the element in global coordinates 
Uprev=Ue; %update Uprev of element for use in next state determination call
%% calculate element deformation increments
[dvax,dvr] = ELDFO2(ddise,fl,cosa,sina);
%% UPDATE AXIAL FORCES AND AXIAL ENERGY
dfax=eal*dvax;      
ftot(1,1)=ftot(1,1)-dfax;
ftot(2,1)=ftot(2,1)+dfax;  
%% MOMENTS IN ELASTIC COMPONENT AT BEGINING OF STEP
bmel(1,1)=bmtot(1,1)-bmep(1,1);
bmel(2,1)=bmtot(2,1)-bmep(2,1);
%% LINEAR MOMENT INCREMENTS FOR ELASTO-PLASTIC COMPONENT - SET IN DBM
[dbm] = BMCAO2(dvr,kody,ek11,ek12,ek22,ek22h,ek11h);
%% TRACE NONLINEAR PATH FOR ELASTO-PLASTIC COMPONENT---state determination
facac=0.0;
while (facac<0.999999)
    factor=1.0-facac;
    % PLASTIC HINGE ROTATIONS
    kod=kody(1,1)+kody(2,1)-1.0;
    if(kod>0)
        % hinges at both ends
        dpr(1,1)=dvr(1,1);
        dpr(2,1)=dvr(2,1);
    elseif(kod==0)
        % hinge at one end only
        dpr(1,1)=dvr(1,1)+pr21*dvr(2,1);
        dpr(2,1)=dvr(2,1)+pr12*dvr(1,1);
    else
         %never executed
    end
         
    % CALCULATE WHICH END HAS NEXT EVENT IF YIELDS, SET KFAC=IEND AND BBMY=YIELD VALUE
    % SET EVENT FACTOR IN FACTOR
    kfac=3;
    for iend=1:2
        if (kody(iend,1)==0.0)
            dbmm=dbm(iend,1);
            % elastic, get factor for status change(no hinge at end)
            if (dbmm<0.0)
                dbmo=bmy(iend,2)-bmep(iend,1);
                if(dbmo>=dbmm) 
                    fac=dbmo/dbmm;
                else
                    fac=2.0;
                end 
                if (fac<=factor)
                    factor=fac;
                    bbmy=bmy(iend,2);
                    kfac=iend;
                end
            elseif(dbmm>0.0)
                dbmo=bmy(iend,1)-bmep(iend,1);
                if(dbmo<=dbmm) 
                    fac=dbmo/dbmm;
                else
                    fac=2.0;
                end 
                if (fac<=factor)
                    factor=fac;
                    bbmy=bmy(iend,1);
                    kfac=iend;
                end
            else
            end
        else
            % hinge at this end
            if(bmep(iend,1)*dpr(iend,1)<0.0)
            % unloading (plastic work negative)
                factor=0.0;
                kfac=0.0;
                kody(iend,1)=0.0;
            else
                % continuing to yield (plastic work positive)
            end
        end
    end
    % UPDATE BENDING STATE AND CALCULATE BENDING ENERGY
    % dbm= elastic increment - use if elastic bbmy= yield value - use if yields
    if(kfac~=0)
        for iend=1:2
            if(iend==kfac)
                % new hinge at this end
                bmep(iend,1)=bbmy;
                kody(iend,1)=1;
            elseif(kody(iend,1)==0)
                % this end remains elastic
                dmep=factor*dbm(iend,1);
                bmep(iend,1)=bmep(iend,1)+dmep;
            else
                % this end remains plastic
                dppr=factor*dpr(iend,1);
                prtot(iend,1)=prtot(iend,1)+dppr;
                if (dppr<0.0)
                    pracn(iend,1)=pracn(iend,1)+dppr;
                else
                    pracp(iend,1)=pracp(iend,1)+dppr;
                end
            end
        end
    else
        % unloads - factor=0.
    end
    % CHECK COMPLETION OF CYCLE
    facac=facac+factor;
    if (facac<0.99999)
        % cycle not completed, calculate new moment increments
        [dbm] = BMCAO2(dvr,kody,ek11,ek12,ek22,ek22h,ek11h);
    end
end
%% YIELD MOMENTS FOR NEXT STEP
if(ksurf==1)
    [bmy] = YMOM02(ftot,pmx,a1,a2,bmy);
    % CHECK YIELD SURFACE OVERSHOOT
    for iend=1:2
        if (kody(iend,1)~=0.0)
        % inelastic on old surface
            if (bmep(iend,1)>bmy(iend,1)) 
                % inelastic positive on new surface also
                bmep(iend,1)=bmy(iend,1);
            elseif (bmep(iend,1)<bmy(iend,2))
                % inelastic negative on new surface also
                bmep(iend,1)=bmy(iend,2);
            elseif ((bmep(iend,1)<(bmy(iend,1)*0.98)) && (bmep(iend,1)>(bmy(iend,2)*0.98)))
                % moves inside new surface by > 2% - reset yield code
                kody(iend,1)=0;
            else
            end
        else
            % elastic on old surface
            if (bmep(iend,1)>bmy(iend,1))
                % inelastic positive on new surface
                bmep(iend,1)=bmy(iend,1);
                kody(iend,1)=1;
            elseif (bmep(iend,1)<=bmy(iend,2))
                % inelastic negative on new surface
                bmep(iend,1)=bmy(iend,2);
                kody(iend,1)=1;
            else
            end
        end
    end
end
%% UPDATE TOTAL FORCES
dsf=(bmtot(1,1)+ bmtot(2,1))/fl;
ppsh=psh/(1.0-psh);
dmeli=(ek11*dvr(1,1)+ek12*dvr(2,1))*ppsh+bmel(1,1);
dmelj=(ek12*dvr(1,1)+ ek22*dvr(2,1))*ppsh+bmel(2,1);
bmtot(1,1)=bmep(1,1)+dmeli;
bmtot(2,1)=bmep(2,1)+dmelj;
dsf=dsf-(bmtot(1,1)+bmtot(2,1))/fl;
sftot(1,1)=sftot(1,1)-dsf;
sftot(2,1)=sftot(2,1)+dsf;

RF = ELASO2(ndof,ftot,cosa,sina,sftot,bmtot);

% Form total restoring force vector
TotalRF = zeros(NumFreeDOF, 1);
    
% Get element nodes to assemble in the structure restoring force vector
if Node1UX <= NumFreeDOF
    TotalRF(Node1UX, 1) = RF(1, 1);
end
if Node1UY <= NumFreeDOF
    TotalRF(Node1UY, 1) = RF(2, 1);
end
if Node1THETA <= NumFreeDOF
    TotalRF(Node1THETA, 1) = RF(3, 1);
end
if Node2UX <= NumFreeDOF
    TotalRF(Node2UX, 1) = RF(4, 1);
end
if Node2UY <= NumFreeDOF
    TotalRF(Node2UY, 1) = RF(5, 1);
end
if Node2THETA <= NumFreeDOF
    TotalRF(Node2THETA, 1) = RF(6, 1);
end





%%%%%%% FUNCTIONS %%%%%%%%%
function [bmy] = YMOM02(ftot,pmx,a1,a2,bmy)
facc=-1.0;
for iend = 1 : 2
    % Change sign of axial force and end 1
    fft = ftot(iend,1) * facc;
    facc = 1;
    fac = 1;
    for j = 1 : 2
        fac = -fac;
        yieldcalc = 0;  % flag if the yield moment is calculated inside 
                        % this next for loop
        for i = 1 : 3
            if (fft < pmx(i,j,iend))
                yieldcalc = 1;  % set flag since the condition was met
                % Calculate yield moment (M = a2 + a1P)
                bbmy = a2(i,j,iend) - a1(i,j,iend) * fft;
                if (fac * bbmy > 0) 
                    % Axial force is beyond Pc and Pt
                    bbmy = 0;
                end
                bmy(iend,j) = bbmy;
            end
        end
        % Only calculate yield moment if it wasn't calculated in the above
        % for loop
        if (yieldcalc == 0)
            i = 4;
            % Calculate yield moment (M = a2 + a1P)
            bbmy = a2(i,j,iend) - a1(i,j,iend) * fft;
            if (fac * bbmy > 0) 
                % Axial force is beyond Pc and Pt
                bbmy = 0;
            end
            bmy(iend,j) = bbmy;
        end
    end
end
%c ---------------------------------INTERCHANGE BMY(1,1) AND BMY(1,2) AND
%c ------------------------------AND ALSO CHANGE SIGN OF MOMENTS AT END 1
fac=-bmy(1,1);
bmy(1,1)=-bmy(1,2);
bmy(1,2)=fac;
      
      
      
      
      
function [dbm] = BMCAO2(dvr,kody,ek11,ek12,ek22,ek22h,ek11h)
dbm=zeros(2,1);
% c ------------------SET KYY TO INDICATE TYPE OF ELEMENT STIFFNESS TO USE
      kyy=kody(1,1)+2*kody(2,1)+1;
      if(kyy==1)
%c---no hinge at either end
        dbm(1,1)=ek11*dvr(1,1)+ek12*dvr(2,1);
        dbm(2,1)=ek12*dvr(1,1)+ek22*dvr(2,1);
      elseif(kyy==2)
%c---hinge at end 1
        dbm(1,1)=0.0;
        dbm(2,1)=ek22h*dvr(2,1);
      elseif(kyy==3)
%c---hinge at end 2
        dbm(1,1)=ek11h*dvr(1,1);
        dbm(2,1)=0.0;
      elseif(kyy==4)
%c---hinges at both end
        dbm(1,1)=0.0;
        dbm(2,1)=0.0;
       else
           %never executed
      end
      
      
      
      
      
      
      
      
      
      
   %%
function [relas] = ELASO2(ndof,ftot,cosa,sina,sftot,bmtot)
%%
relas=zeros(ndof,1);
%BASIC RESISTING FORCES
      relas(1,1)=(ftot(1,1)-0)*cosa-(sftot(1,1)-0)*sina;
      relas(2,1)=(ftot(1,1)-0)*sina+(sftot(1,1)-0)*cosa;
      relas(3,1)=bmtot(1,1)-0-0;
      relas(4,1)=(ftot(2,1)-0)*cosa-(sftot(2,1)-0)*sina;
      relas(5,1)=(ftot(2,1)-0)*sina+(sftot(2,1)-0)*cosa;
      relas(6,1)=bmtot(2,1)-0-0;
%%







%%
function [dvax,dvr] = ELDFO2(ddise,f1,cosa, sina) 
%%
dvr=zeros(2,1);
%DEFORMATION INCREMENTS OR DEFORMATION RATES
      dvax=cosa*(ddise(4,1)-ddise(1,1))+sina*(ddise(5,1)-ddise(2,1));
      rot=(sina*(ddise(4,1)-ddise(1,1))+cosa*(ddise(2,1)-ddise(5,1)))/f1;
      dvr(1,1)=ddise(3,1)+rot;
      dvr(2,1)=ddise(6,1)+rot;
%%
